simulink library "formationFlyingBlockset"  (R2016b)
settings: Solver=ode45  StartTime=0.0  StopTime=10.0  RelTol=1e-3  EnableMultiTasking=on
undefined symbols (not defined in the file or in its folder): adaptive, aircraftmask_ID, aircraftmask_navigationLaw, aircraftmask_originNED_ECEF_rrm, aircraftmask_p0_NED_m, aircraftmask_phithetapsi_trim, aircraftmask_wakevortexenabled, airkraftmask_displayLeader, DiscIntNeverNeededParam, Earth, fflib_degdegm2rrm, fflib_Hz2radps, fflib_rrm2degdegm, flat2lla, hinf, Klqr, lquadr, mask_ac, mask_ID, mpc, poleplacement, uavsim, washout, WGS84
undefined symbols (not defined in the file): aircraftmask_phithetapsi0, aircraftmask_pqr0, aircraftmask_uvw0, innerloop, outerloop, tatestos
libraries: formationFlyingBlockset x59, aerolibtransform2 x42, simulink_extras x27, dspsrcs4 x11, aerolibutil x5, uavsimBlockset_UAV3DInterface x4, uavsimBlockset_ServoHS55 x4, uavsimBlockset_VectorNorm x3, uavsimBlockset_UAV3DVisualization x3, uavsimBlockset_AugmentWind x3, stringquartett x2, Parrot_DCAS_lib x2
(part 1 of 5)
settings Model: Creator=j.bolting  LastModifiedBy=j.bolting
settings DataIOCC: LimitDataPoints=on  SaveFormat=Array
settings OptimizationCC: ExpressionDepthLimit=2147483647  LifeSpan=inf
settings DebuggingCC: UnderspecifiedInitializationDetection=Classic  MergeDetectMultiDrivingBlocksExec=none  SolverPrmCheckMsg=warning  AllowSymbolicDim=off  StateNameClashWarn=warning  SFUnexpectedBacktrackingDiag=warning  SFNoUnconditionalDefaultTransitionDiag=warning  SFExecutionAtInitializationDiag=none
settings HardwareCC: ProdBitPerPointer=32  ProdBitPerSizeT=32  ProdBitPerPtrDiffT=32  ProdLargestAtomicFloat=None  ProdIntDivRoundTo=Undefined  ProdEndianess=Unspecified  ProdWordSize=32  ProdHWDeviceType=32-bit Generic
settings ModelReferenceCC: PropagateSignalLabelsOutOfModel=off
settings GRTTargetCC: TargetLangStandard=C89/C90 (ANSI)  GeneratePreprocessorConditionals=Disable all
settings ConfigComp: CovMetricSettings=dw  CovHtmlReporting=on  CovSaveCumulativeToWorkspaceVar=on  CovSaveSingleToWorkspaceVar=on  CovExternalEMLEnable=off  CovSFcnEnable=off

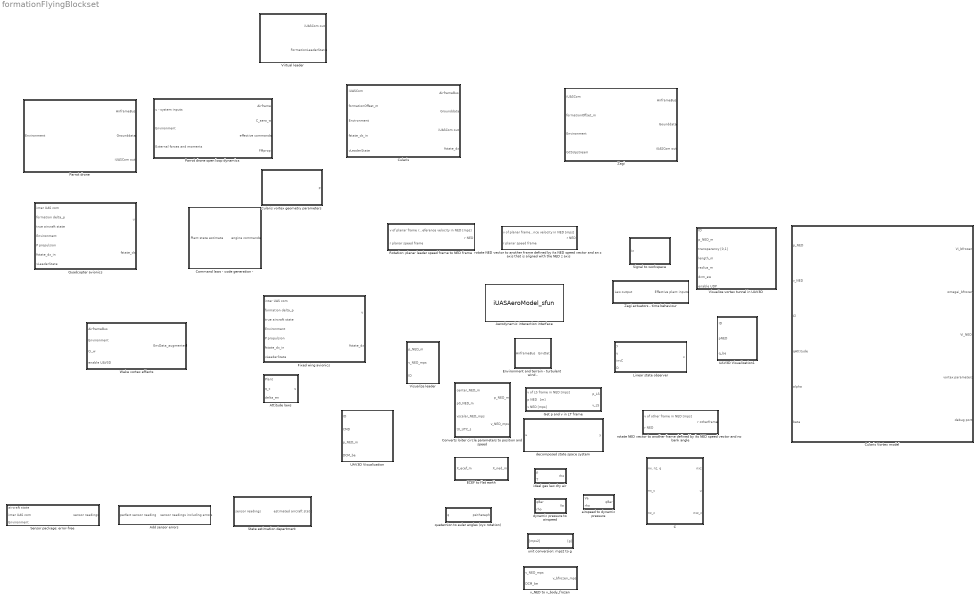
== system formationFlyingBlockset ==
  Add sensor errors : Subsystem
  Aerodynamic interaction interface : M-S-Function  FunctionName=iUASAeroModel_sfun  Parameters=mask_ID, mask_c_m, mask_wingspan_m, mask_sweepangle_rad, mask_dihedral_rad, mask_l_longi_m, mask_nosecoo_m, mask_l_vertical_m, mask_fincoo_m  mask{mask_c_m=0, mask_ID=0, mask_wingspan_m=0, mask_sweepangle_rad=0, mask_dihedral_rad=0, mask_l_longi_m=0, mask_nosecoo_m=0, mask_l_vertical_m=0, mask_fincoo_m=0}
      mask prompts: mask_c_m "Mean aerodynamic chord [m]"; mask_ID "Aircraft ID"; mask_wingspan_m "Wingspan"; mask_sweepangle_rad "Wing sweep angle [rad]"; mask_dihedral_rad "Wing dihedral angle [rad]"; mask_l_longi_m "Longitudinal reference length [m], typically the length of the fuselage"; mask_nosecoo_m "Nose coordinates in the body frame [m m m]"; mask_l_vertical_m "Vertical reference length [m], typically the distance between the lowest point of the fuselage and the tip of the vertical stabilizer"; mask_fincoo_m "Fin tip coordinates in the body frame [m m m]"
      mask help:
      | Interface to the aerodynamic interaction model.
      | This block computes the induced velocities and
      | rotation rates caused by other close UAS and,
      | at the same time, communicates the state of the
      | UAS connected to this block to the aerodynamic
      | interaction model to build a list of all UASs
      | in the airspace.
      mask Display:
      | % Input port names:
      | port_label('input',1,'p{NED}','texmode','on');
      | port_label('input',2,'v{NED}','texmode','on');
      | port_label('input',3,'C_L','texmode','on');
      | port_label('input',4,'q_{Attitude}','texmode','on');
      | port_label('input',5,'[\alpha, \beta]','texmode','on');
      | 
      | % output port names
      | port_label('output',1,'V_{i}^{bfrozen}','texmode','on');
      | port_label('output',2,'\omega_{i}^{bfrozen}','texmode','on');
      | port_label('output',3,'V_i^{NED}','texmode','on');
  Attitude laws : Subsystem  SystemSampleTime=uavsim.ap.hardware.dt_attitudeloops_s
  C : Subsystem
  Command laws - code generation - : Subsystem  TreatAsAtomicUnit=on  SystemSampleTime=0.01
  Converts loiter circle parameters to position and speed : Subsystem
  Cularis : Subsystem  mask{aircraftmask_phithetapsi0=[uavsim.cularis.phithetapsi0(1:2); deg2rad(-30)]', aircraftmask_p0_NED_m=[0 0 -50], aircraftmask_originNED_ECEF_rrm=uavsim.originNED_ECEF_radradm, aircraftmask_pqr0=uavsim.cularis.omega0, aircraftmask_uvw0=uavsim.cularis.uvw0, aircraftmask_phithetapsi_trim=uavsim.cularis.phithetapsi0, aircraftmask_ID=1, aircraftmask_wakevortexenabled=off, aircraftmask_navigationLaw=2, uavsim=uavsim, leaderID=0, airkraftmask_displayLeader=on}
      mask prompts: aircraftmask_phithetapsi0 "Initial Euler angles [rad]"; aircraftmask_p0_NED_m "Initial position, NED frame [m]"; aircraftmask_originNED_ECEF_rrm "Origin NED frame. ECEF, [rad rad m]"; aircraftmask_pqr0 "Initial rotation rates, body frame [rad/s]"; aircraftmask_uvw0 "Initial velocity, body frame [m/s]"; aircraftmask_phithetapsi_trim "Trim Euler angles [rad]"; aircraftmask_ID "Aircraft ID"; aircraftmask_wakevortexenabled "Wake vortex interaction enabled"; aircraftmask_navigationLaw "Active navigation law (-1: automatic selection)"; uavsim "Parameter set"; leaderID "Follows which ID?"; airkraftmask_displayLeader "Display virtual leader"
      mask Display:
      | % Set Icon:
      | image(imread('images/cularis.png'), [.2, .2, .6, .6])
  Cularis Vortex model : Subsystem  mask{mask_ID=aircraftmask_ID}
      mask prompts: mask_ID "ID"
  Cularis vortex geometry parameters : Subsystem  mask{mask_ID=mask_ID}
      mask prompts: mask_ID "ID"
  ECEF to flat earth : Subsystem  mask{mask_originNED_ECEF_rrm=aircraftmask_originNED_ECEF_rrm}
      mask prompts: mask_originNED_ECEF_rrm "Origin NED (lat lon alt [rad, rad, m])"
  Environment and terrain - turbulent wind - : Subsystem  mask{mask_ambientWind=uavsim.environment.ambientWind_NED_mps, mask_wingspan=uavsim.cularis.b, mask_turbulenceON=off, mask_windON=off}
      mask prompts: mask_ambientWind "Ambient wind vector, NED [m/s]"; mask_wingspan "Aircraft wing span [m]"; mask_turbulenceON "Turbulence ON?"; mask_windON "Ambient wind ON?"
  Fixed wing avionics : Subsystem  mask{mask_ac=uavsim.cularis}
      mask prompts: mask_ac "Aircraft specific structure"
      mask Display: image(imread('images/avionics.png'),[.3, .3, .4, .4])
  Get p and v in LT frame : Subsystem
  Linear state observer : Subsystem
  Parrot drone : Subsystem  mask{aircraftmask_phithetapsi0=[uavsim.cularis.phithetapsi0(1:2); deg2rad(-30)]', aircraftmask_p0_NED_m=[0 0 -50], aircraftmask_originNED_ECEF_rrm=uavsim.originNED_ECEF_radradm, aircraftmask_pqr0=uavsim.cularis.omega0, aircraftmask_uvw0=uavsim.cularis.uvw0, aircraftmask_phithetapsi_trim=uavsim.cularis.phithetapsi0, aircraftmask_ID=1, aircraftmask_wakevortexenabled=off, aircraftmask_navigationLaw=2, uavsim=uavsim, leaderID=0, airkraftmask_displayLeader=on}
      mask prompts: aircraftmask_phithetapsi0 "Initial Euler angles [rad]"; aircraftmask_p0_NED_m "Initial position, NED frame [m]"; aircraftmask_originNED_ECEF_rrm "Origin NED frame. ECEF, [rad rad m]"; aircraftmask_pqr0 "Initial rotation rates, body frame [rad/s]"; aircraftmask_uvw0 "Initial velocity, body frame [m/s]"; aircraftmask_phithetapsi_trim "Trim Euler angles [rad]"; aircraftmask_ID "Aircraft ID"; aircraftmask_wakevortexenabled "Wake vortex interaction enabled"; aircraftmask_navigationLaw "Active navigation law (-1: automatic selection)"; uavsim "Parameter set"; leaderID "Follows which ID?"; airkraftmask_displayLeader "Display virtual leader"
      mask Display:
      | % Set Icon:
      | image(imread('images/parrot.png'), [.2, .2, .6, .6])
  Parrot drone open loop dynamics : Subsystem  mask{mask_phithetapsi0=aircraftmask_phithetapsi0, mask_p0_ECEF_lla=fflib_degdegm2rrm(flat2lla(aircraftmask_p0_NED_m, rad2deg(aircraftmask_originNED_ECEF_rrm(1:2)), 0, aircraftmask_originNED_ECEF_rrm(3))), mask_originNED_ECEF_rrm=aircraftmask_originNED_ECEF_rrm, mask_pqr0=aircraftmask_pqr0, mask_uvw0=aircraftmask_uvw0, uavsim=uavsim}
      mask prompts: mask_phithetapsi0 "Initial euler angles [rad]"; mask_p0_ECEF_lla "Initial position ECEF [rad rad m]"; mask_originNED_ECEF_rrm "Origin NED frame, ECEF-WGS84, [rad rad m]"; mask_pqr0 "Initial body rotation rates [rad/s]"; mask_uvw0 "Initial velocity body frame [m/s]"; uavsim "Parameter set"
      mask Display: image(imread('images/parrot.png'),[.3, .3, .4, .4])
  Quadcopter avionics : Subsystem  mask{mask_ac=uavsim.parrot}
      mask prompts: mask_ac "Aircraft specific structure"
      mask Display: image(imread('images/avionics.png'),[.3, .3, .4, .4])
  Rotation: planar leader speed frame to NED frame : Subsystem
  Sensor package: error-free : Subsystem
  Signal to workspace : Subsystem  InitFcn=|  mask{mask_id=['log_ucontroller_UAS' num2str(aircraftmask_ID) '_Signalname'], mask_dt=-1, mask_debug=tatestos}
      | twblock = find_system(gcb, 'LookUnderMasks', 'all' ,'FollowLinks','on', 'BlockType', 'ToWorkspace' );
      | maskblock = find_system(gcb);
      | % Disable library link to be able to modify the block
      | set_param(maskblock{1}, 'LinkStatus', 'inactive');
      | maskparams = get_param(maskblock, 'MaskValues');
      | id = maskparams{1}{3};
      | set_param(twblock{1}, 'VariableName', id);
      | set_param(twblock{1}, 'Name', id);
      mask prompts: mask_id "Variable ID [string, char array], e.g. 'log_voltage'"; mask_dt "Sample time [s]"; mask_debug "debug value"
      mask init:
      | mask_ida = mask_id;
      | mv = get_param(gcb, 'MaskValues');
      | mv{3} = mask_ida;
      | set_param(gcb, 'MaskValues', mv);
      settings: PostSaveFcn=|
      | maskblock = find_system(gcb);
      | set_param(maskblock{1}, 'LinkStatus', 'restore')
      mask Display:
      | % Set Icon:
      | image(imread('images/blocklogo_datalogger.png'))
  State estimation department : Subsystem
  UAV3D Visualization : Subsystem  TreatAsAtomicUnit=on  SystemSampleTime=uavsim.ap.hardware.dt_navigationloops_s  mask{mask_visual=0}
      mask prompts: mask_visual "3D model"
      mask TypeOptions mask_visual: 0 | 1 | 2 | 3
  UAV3D Visualization1 : Subsystem  TreatAsAtomicUnit=on  SystemSampleTime=uavsim.simConfig.tsample_UAV3D  mask{mask_visual=2}
      mask prompts: mask_visual "3D model"
      mask TypeOptions mask_visual: 0 | 1 | 2 | 3
  Virtual leader : Subsystem  mask{aircraftmask_originNED_ECEF_rrm=uavsim.originNED_ECEF_radradm, aircraftmask_ID=0, uavsim=uavsim}
      mask prompts: aircraftmask_originNED_ECEF_rrm "Origin NED frame. ECEF, [rad rad m]"; aircraftmask_ID "Aircraft ID"; uavsim "Parameter set"
      mask Display:
      | % Set Icon:
      | image(imread('images/cularis.png'), [.2, .2, .6, .6])
  Visualize leader : Subsystem  TreatAsAtomicUnit=on  SystemSampleTime=uavsim.simConfig.tsample_UAV3D  mask{mask_3dmodel=1}
      mask prompts: mask_3dmodel "3D model"
      mask TypeOptions mask_3dmodel: 0 | 1 | 2 | 3
  Visualize vortex tunnel in UAV3D : Subsystem  TreatAsAtomicUnit=on  SystemSampleTime=uavsim.simConfig.tsample_UAV3D
  Wake vortex effects : Subsystem  TreatAsAtomicUnit=on
  Zagi : Subsystem  mask{aircraftmask_phithetapsi0=[uavsim.zagi.phithetapsi0(1:2); deg2rad(30)]', aircraftmask_p0_NED_m=[0 0 -50], aircraftmask_originNED_ECEF_rrm=uavsim.originNED_ECEF_radradm, aircraftmask_pqr0=uavsim.zagi.omega0, aircraftmask_uvw0=uavsim.zagi.uvw0, aircraftmask_phithetapsi_trim=uavsim.zagi.phithetapsi0, aircraftmask_ID=1, aircraftmask_wakevortexenabled=off, aircraftmask_navigationLaw=3, uavsim=uavsim, leaderID=0}
      mask prompts: aircraftmask_phithetapsi0 "Initial Euler angles [rad]"; aircraftmask_p0_NED_m "Initial position, NED frame [m]"; aircraftmask_originNED_ECEF_rrm "Origin NED frame. ECEF, [rad rad m]"; aircraftmask_pqr0 "Initial rotation rates, body frame [rad/s]"; aircraftmask_uvw0 "Initial velocity, body frame [m/s]"; aircraftmask_phithetapsi_trim "Trim Euler angles [rad]"; aircraftmask_ID "Aircraft ID"; aircraftmask_wakevortexenabled "Wake vortex interaction enabled"; aircraftmask_navigationLaw "Active navigation law (-1: automatic selection)"; uavsim "Parameter set"; leaderID "Follows which ID?"
      mask Display:
      | % Set Icon:
      | image(imread('images/zagi_slope.png'))
      | %image(imread('images/aerosonde_MKII.png'),[.2, .2, .6, .6])
      | % Port labels:
      | port_label('input',1,'Com_{interUAS}','texmode','on');
      | port_label('input',2,'offset_{formation}','texmode','on');
      | port_label('input',3,'Environment','texmode','on');
      | port_label('input',4,'GCS_{Upstream}','texmode','on');
      | 
      | port_label('output',1,'Airframe_{Bus}','texmode','on');
      | port_label('output',2,'GroundData','texmode','on');
      | port_label('output',3,'iUAS_{Com}','texmode','on');
  Zagi actuators - time behaviour : Subsystem  TreatAsAtomicUnit=on
  airspeed to dynamic pressure : Subsystem
  decomposed state space system : Subsystem  mask{ss_innerloop=innerloop, ss_outerloop=outerloop}
      mask prompts: ss_innerloop "State space model inner loop"; ss_outerloop "State space model outer loop"
  dynamic pressure to airspeed : Subsystem
  ideal gas law dry air : Subsystem
  quaternion to euler angles (zyx rotation) : Subsystem
  rotate NED vector to another frame defined by its NED speed vector and an z axis that is aligned with the NED z axis : Subsystem
  rotate NED vector to another frame defined by its NED speed vector and no bank angle : Subsystem
  unit conversion: mps2 to g : Subsystem
  v_NED to v_body_frozen : Subsystem

== system formationFlyingBlockset/Add sensor errors ==
  perfect sensor reading : Inport  OutDataTypeStr=Bus: SensorBus
  AHRS : Subsystem
  Air Data : Subsystem
  Bus Object Bus Creator : BusCreator  Inputs=8  OutDataTypeStr=Bus: SensorBus  mask(BUS OBJECT Bus Creator){busType=Bus: SensorBus}
      mask prompts: busType "Bus Type"
      mask help:
      | Provides users the cabability to painlessly, instantly customize bus creators of output data type 'Bus:' by selecting the bus object type from a drop down menu dynamically populated by bus objects in the workspace.
      |
      | After pressing the "Apply Selection" button signal lines into the creator are populated and named with the elements in the chosen bus saving the user from having to recall and fill out signal line names.
      |
      | NOTE that when copying a Bus Object Bus Creator from your locked Library the link to the Library is automatically broken. This saves the user from having to Unlock Links To Library (From the Library menu.), Disable Link and finally Break Link (Both from the Model menu.) for every placed instance of the block.
      settings: AttributesFormatString=%<OutDataTypeStr>  CopyFcn=set_param(gcb, 'LinkStatus', 'none')
      mask TypeOptions busType: Bus: AHRS | Bus: Acceleration | Bus: Aero | Bus: Airdata | Bus: Airframe | Bus: Attitude | Bus: CMD | Bus: CMD_quadrotor | Bus: ControlInfoBus | Bus: Enginedata | Bus: Environment | Bus: FlightGearData | Bus: GCSUpstream | Bus: GNSSL1 | Bus: GNSSRTK | Bus: GPS | Bus: IMU | Bus: Kinematics | Bus: LandinggearInput | Bus: MotionTracker | Bus: Position | Bus: Radiodistance | Bus: RotationalAcceleration | Bus: RotationalVelocity | Bus: SensorBus | Bus: StateBus | Bus: Velocity | Bus: WindAngles | Bus: iUAScom
      mask Callback busType:
      | % Using variable names terminated with "_BOBC" to lessen the chances of
      | % collisions with existing workspace variables.
      | 
      | % Get the current block handle and mask handle.
      | handleCreator_BOBC = gcbh;
      | maskObj_BOBC       = Simulink.Mask.get(gcb);
      | 
      | % Get a list of variables in the workspace in order to search for the '1x1
      | % Bus' types.
      | wsVars_BOBC = whos;
      | 
      | % Reset the 'TypeOptions' bus list in case some '1x1 Bus' types have been
      | % deleted from or added to the workspace.
      | maskObj_BOBC.Parameters.TypeOptions = {'<empty>'};
      | 
      | % Reset the bus count.
      | busCount_BOBC = 0;
      | 
      | for index_BOBC = 1:length(wsVars_BOBC)
      | 
      |    % If the variable is a bus object...
      |    if strcmp(wsVars_BOBC(index_BOBC).class, 'Simulink.Bus')
      | 
      |       busCount_BOBC = busCount_BOBC + 1;
      | 
      |       % ... add it to the TypeOptions of the mask.
      |       maskObj_BOBC.Parameters.TypeOptions(busCount_BOBC) = ...
      |                                                            ...
      |                                  {['Bus: ', wsVars_BOBC(index_BOBC).name]};
      |    end
      | end
      | 
      | if busCount_BOBC == 0
      | 
      |    % If there are NO bus objects in the workspace then provide a warning
      |    % popup...
      |    warndlg('There are currently no bus objects in the workspace - you have no use for this block. Use a normal Bus Creator instead.')
      | 
      |    % ... and do nothing.
      | elseif ~strcmp(get_param(handleCreator_BOBC, 'OutDataTypeStr'), 'Inherit: auto')
      | 
      |    % If the currently selected bus data type ('OutDataTypeStr') is not
      |    % 'Inherit: auto' (i.e., if we are reopening the mask.) then get the
      |    % current 'OutDataTypeStr' and 'maskVal.' ('maskVal' is the selected
      |    % 'TypeOptions' list member.)
      |    outDatStr_BOBC = get_param(handleCreator_BOBC, 'OutDataTypeStr');
      |    maskVal_BOBC   = get_param(handleCreator_BOBC, 'MaskValues');
      | 
      |    if ~strcmp(outDatStr_BOBC, maskVal_BOBC{1})
      | 
      |       % Upon re-opening the mask if the default 'TypeOptions' list member
      |       % (The first one.) contained in 'maskVal' does not match the
      |       % currently selected bus data type ('OutDataTypeStr') then set the
      |       % 'TypeOptions' list member to the selected bus data type. (Cuts down
      |       % on confusion to have the displayed list member match the selected
      |       % bus data type rather than the first entry.)
      |       set_param(handleCreator_BOBC, 'MaskValues', {outDatStr_BOBC});
      |    end
      | end
      | 
      | % Clean up the workspace.
      | clear  handleCreator_BOBC  maskObj_BOBC     wsVars_BOBC ...
      |             busCount_BOBC    index_BOBC  outDatStr_BOBC ...
      |              maskVal_BOBC
      mask DialogControl applyMOCBSelection Prompt: Apply Selection
      mask DialogControl applyMOCBSelection Callback:
      | % Using variable names terminated with "_BOBC" to lessen the chances of
      | % collisions with existing workspace variables.
      | 
      | % Get the current block, current block handle and mask handle.
      | currentBlock_BOBC  = gcb;
      | handleCreator_BOBC = gcbh;
      | 
      | % Get the desired bus type...
      | desiredBusType_BOBC = get_param(handleCreator_BOBC, 'busType');
      | 
      | % ... and set the 'OutDataTypeStr' to it.
      | set_param(handleCreator_BOBC, 'OutDataTypeStr', desiredBusType_BOBC);
      | 
      | %% First delete any existing lines on the port.
      | % Get the line handles.
      | lh_BOBC = get_param(handleCreator_BOBC, 'LineHandles');
      | 
      | % If any lines exist (Non- -1 line handles.), delete them and start over.
      | if max(lh_BOBC.Inport > 0)
      | 
      |    for index_BOBC = 1:length(lh_BOBC.Inport)
      | 
      |       if lh_BOBC.Inport(index_BOBC) > 0
      | 
      |          delete_line(lh_BOBC.Inport(index_BOBC))
      |       end
      |    end
      | end
      | 
      | %% Then work on adding new lines.
      | 
      | % Get the block path for 'add_line' function.
      | blockPath_BOBC = get_param(handleCreator_BOBC, 'Parent');
      | 
      | % Get the newly selected bus type ('OutDataTypeStr')...
      | mocbBusType_BOBC = get_param(currentBlock_BOBC, 'OutDataTypeStr');
      | 
      | % ... and parse off "Bus: " so the string of the desired bus contained in
      | % 'OutDataTypeStr' matches the raw workspace bus names.
      | mocbBusType_BOBC = mocbBusType_BOBC(6:end);
      | 
      | % Then evaluate the string containing the workspace bus name which will
      | % load the desired bus parameters.
      | busParams_BOBC = eval(mocbBusType_BOBC);
      | 
      | % From the parameters grab the number of lines to add.
      | numLines_BOBC = length(busParams_BOBC.Elements);
      | 
      | % Set the number of inputs of the masked bus creator to the number of lines
      | % to add.
      | set_param(handleCreator_BOBC, 'Inputs', num2str(numLines_BOBC));
      | 
      | % Get (Inputs.) port handles so we can grab the positions of them.
      | ph_BOBC = get_param(handleCreator_BOBC, 'PortHandles');
      | 
      | for index_BOBC = 1:numLines_BOBC
      | 
      |    % Get the position of input port number 'index_BOBC'.
      |    portPos_BOBC = get_param(ph_BOBC.Inport(index_BOBC), 'Position');
      | 
      |    % Add a line from 50 pixels left of the port position to the port
      |    % position. (This must be done because it's the lines that get named,
      |    % not the port positions.)
      |    portLine_BOBC = add_line(blockPath_BOBC, [portPos_BOBC - [50 0]; portPos_BOBC]);
      | 
      |    % Rename the new line to the bus 'index_BOBC-st/nd/rd/th' element name.
      |    set_param(portLine_BOBC, 'Name', busParams_BOBC.Elements(index_BOBC).Name)
      | end
      | 
      | %% Cleanup the workspace.
      | clear    currentBlock_BOBC  handleCreator_BOBC      index_BOBC ...
      |        desiredBusType_BOBC             lh_BOBC  blockPath_BOBC ...
      |           mocbBusType_BOBC      busParams_BOBC   numLines_BOBC ...
      |                    ph_BOBC        portPos_BOBC   portLine_BOBC
  L1 GPS : Subsystem
  Optitrack : Subsystem
  Propulsion sensors : Subsystem
  RTK DGPS : Subsystem
  Radio distance sensor : Subsystem
  Wind angle sensors : Subsystem
  sensor readings including errors : Outport  OutDataTypeStr=Bus: SensorBus
  wires:
  Bus Object Bus Creator/1 -> sensor readings including errors/1
  perfect sensor reading/1 -> AHRS/1(perfect sensor reading), RTK DGPS/1(perfect sensor reading), L1 GPS/1(perfect sensor reading), Optitrack/1(perfect sensor reading), Propulsion sensors/1(perfect sensor reading), Radio distance sensor/1(perfect sensor reading), Wind angle sensors/1(perfect sensor reading), Air Data/1(perfect sensor reading)
  AHRS/1(output) -> Bus Object Bus Creator/1  "ahrs"
  Air Data/1(output) -> Bus Object Bus Creator/2  "airdata"
  L1 GPS/1(output) -> Bus Object Bus Creator/3  "gnss_l1"
  RTK DGPS/1(output) -> Bus Object Bus Creator/4  "gnss_rtk"
  Propulsion sensors/1(output) -> Bus Object Bus Creator/5  "propulsion"
  Radio distance sensor/1(output) -> Bus Object Bus Creator/6  "radiodistance"
  Wind angle sensors/1(output) -> Bus Object Bus Creator/7  "windangles"
  Optitrack/1(output) -> Bus Object Bus Creator/8  "motiontracker"

== system formationFlyingBlockset/Attitude laws ==
  Plant : Inport  OutDataTypeStr=Bus: StateBus
  q_c : Inport  Port=2
  delta_en : Inport  Port=3
  Add : Sum
  Add1 : Sum
  Bus Creator2 : BusCreator  Inputs=5  OutDataTypeStr=Bus: CMD  NonVirtualBus=on
  Constant : Constant  Value=zeros(3,1)
  Demux : Demux
  Local rotation angle attitude control : Subsystem
  Mux : Mux  Inputs=2
  Saturation : Saturate  UpperLimit=1  LowerLimit=0
  Trim Inputs : Constant  Value=[mask_ac.u_trim(1:4)]
  no flaps : Constant  Value=0
  u : Outport  OutDataTypeStr=Bus: CMD
  wires:
  Demux/4 -> Saturation/1  "den_0to1"
  Local rotation angle attitude control/1(u) -> Add1/1
  Bus Creator2/1 -> u/1  "CMD"
  Demux/3 -> Bus Creator2/3  "dr_rad"
  Saturation/1 -> Bus Creator2/4  "den_0to1"
  Demux/1 -> Bus Creator2/1  "da_rad"
  Demux/2 -> Bus Creator2/2  "de_rad"
  Trim Inputs/1 -> Add/1
  Add/1 -> Demux/1
  Plant/1 -> Local rotation angle attitude control/1(Plant)
  q_c/1 -> Local rotation angle attitude control/2(q_c)
  Constant/1 -> Mux/1
  Mux/1 -> Add1/2
  Add1/1 -> Add/2
  delta_en/1 -> Mux/2
  no flaps/1 -> Bus Creator2/5  "df_rad"

== system formationFlyingBlockset/C ==
  "nx, nz, q" : Inport
  nx_c : Inport  Port=2
  nz_c : Inport  Port=3
  Gain1 : Gain  Gain=Klqr  Multiplication=Matrix(K*u)
  Integrator : Integrator
  Integrator1 : Integrator
  Mux1 : Mux  Inputs=3
  Mux2 : Mux  Inputs=2
  Mux5 : Mux  Inputs=2
  Sum : Sum  Inputs=|+-
  get n_xz : Selector  InputPortWidth=3  IndexOptions=Index vector (dialog)  Indices=1:2  OutputSizes=1
  get q : Selector  InputPortWidth=3  IndexOptions=Index vector (dialog)  Indices=3  OutputSizes=1
  nxz : Outport
  u : Outport  Port=2
  nxz_c : Outport  Port=3
  wires:
  Integrator1/1 -> Mux1/3  "integrated load factor errors"
  nz_c/1 -> Mux2/2
  get q/1 -> Mux5/2
  nx_c/1 -> Mux2/1
  get n_xz/1 -> Sum/1, nxz/1
  Mux2/1 -> Sum/2, nxz_c/1
  Mux5/1 -> Mux1/1
  Sum/1 -> Mux5/1, Integrator1/1  "load factor errors"
  "nx, nz, q"/1 -> get q/1, get n_xz/1
  Gain1/1 -> Integrator/1
  Integrator/1 -> Mux1/2, u/1
  Mux1/1 -> Gain1/1

== system formationFlyingBlockset/Command laws - code generation - ==
  Plant state estimate : Inport  OutDataTypeStr=Bus: StateBus
  Add : Sum  Inputs=+++
  Bus Object Bus Creator : BusCreator  Inputs=1  OutDataTypeStr=Bus: CMD_quadrotor  mask(BUS OBJECT Bus Creator){busType=Bus: CMD_quadrotor}
      mask prompts: busType "Bus Type"
      mask help:
      | Provides users the cabability to painlessly, instantly customize bus creators of output data type 'Bus:' by selecting the bus object type from a drop down menu dynamically populated by bus objects in the workspace.
      |
      | After pressing the "Apply Selection" button signal lines into the creator are populated and named with the elements in the chosen bus saving the user from having to recall and fill out signal line names.
      |
      | NOTE that when copying a Bus Object Bus Creator from your locked Library the link to the Library is automatically broken. This saves the user from having to Unlock Links To Library (From the Library menu.), Disable Link and finally Break Link (Both from the Model menu.) for every placed instance of the block.
      settings: AttributesFormatString=%<OutDataTypeStr>  CopyFcn=set_param(gcb, 'LinkStatus', 'none')
      mask TypeOptions busType: Bus: AHRS | Bus: Acceleration | Bus: Aero | Bus: Airdata | Bus: Airframe | Bus: Attitude | Bus: CMD | Bus: CMD_quadrotor | Bus: ControlInfoBus | Bus: Enginedata | Bus: Environment | Bus: FlightGearData | Bus: GCSUpstream | Bus: GNSSL1 | Bus: GNSSRTK | Bus: GPS | Bus: IMU | Bus: Kinematics | Bus: LandinggearInput | Bus: MotionTracker | Bus: Position | Bus: Radiodistance | Bus: RotationalAcceleration | Bus: RotationalVelocity | Bus: SensorBus | Bus: StateBus | Bus: Velocity | Bus: WindAngles | Bus: iUAScom
      mask Callback busType:
      | % Using variable names terminated with "_BOBC" to lessen the chances of
      | % collisions with existing workspace variables.
      | 
      | % Get the current block handle and mask handle.
      | handleCreator_BOBC = gcbh;
      | maskObj_BOBC       = Simulink.Mask.get(gcb);
      | 
      | % Get a list of variables in the workspace in order to search for the '1x1
      | % Bus' types.
      | wsVars_BOBC = whos;
      | 
      | % Reset the 'TypeOptions' bus list in case some '1x1 Bus' types have been
      | % deleted from or added to the workspace.
      | maskObj_BOBC.Parameters.TypeOptions = {'<empty>'};
      | 
      | % Reset the bus count.
      | busCount_BOBC = 0;
      | 
      | for index_BOBC = 1:length(wsVars_BOBC)
      | 
      |    % If the variable is a bus object...
      |    if strcmp(wsVars_BOBC(index_BOBC).class, 'Simulink.Bus')
      | 
      |       busCount_BOBC = busCount_BOBC + 1;
      | 
      |       % ... add it to the TypeOptions of the mask.
      |       maskObj_BOBC.Parameters.TypeOptions(busCount_BOBC) = ...
      |                                                            ...
      |                                  {['Bus: ', wsVars_BOBC(index_BOBC).name]};
      |    end
      | end
      | 
      | if busCount_BOBC == 0
      | 
      |    % If there are NO bus objects in the workspace then provide a warning
      |    % popup...
      |    warndlg('There are currently no bus objects in the workspace - you have no use for this block. Use a normal Bus Creator instead.')
      | 
      |    % ... and do nothing.
      | elseif ~strcmp(get_param(handleCreator_BOBC, 'OutDataTypeStr'), 'Inherit: auto')
      | 
      |    % If the currently selected bus data type ('OutDataTypeStr') is not
      |    % 'Inherit: auto' (i.e., if we are reopening the mask.) then get the
      |    % current 'OutDataTypeStr' and 'maskVal.' ('maskVal' is the selected
      |    % 'TypeOptions' list member.)
      |    outDatStr_BOBC = get_param(handleCreator_BOBC, 'OutDataTypeStr');
      |    maskVal_BOBC   = get_param(handleCreator_BOBC, 'MaskValues');
      | 
      |    if ~strcmp(outDatStr_BOBC, maskVal_BOBC{1})
      | 
      |       % Upon re-opening the mask if the default 'TypeOptions' list member
      |       % (The first one.) contained in 'maskVal' does not match the
      |       % currently selected bus data type ('OutDataTypeStr') then set the
      |       % 'TypeOptions' list member to the selected bus data type. (Cuts down
      |       % on confusion to have the displayed list member match the selected
      |       % bus data type rather than the first entry.)
      |       set_param(handleCreator_BOBC, 'MaskValues', {outDatStr_BOBC});
      |    end
      | end
      | 
      | % Clean up the workspace.
      | clear  handleCreator_BOBC  maskObj_BOBC     wsVars_BOBC ...
      |             busCount_BOBC    index_BOBC  outDatStr_BOBC ...
      |              maskVal_BOBC
      mask DialogControl applyMOCBSelection Prompt: Apply Selection
      mask DialogControl applyMOCBSelection Callback:
      | % Using variable names terminated with "_BOBC" to lessen the chances of
      | % collisions with existing workspace variables.
      | 
      | % Get the current block, current block handle and mask handle.
      | currentBlock_BOBC  = gcb;
      | handleCreator_BOBC = gcbh;
      | 
      | % Get the desired bus type...
      | desiredBusType_BOBC = get_param(handleCreator_BOBC, 'busType');
      | 
      | % ... and set the 'OutDataTypeStr' to it.
      | set_param(handleCreator_BOBC, 'OutDataTypeStr', desiredBusType_BOBC);
      | 
      | %% First delete any existing lines on the port.
      | % Get the line handles.
      | lh_BOBC = get_param(handleCreator_BOBC, 'LineHandles');
      | 
      | % If any lines exist (Non- -1 line handles.), delete them and start over.
      | if max(lh_BOBC.Inport > 0)
      | 
      |    for index_BOBC = 1:length(lh_BOBC.Inport)
      | 
      |       if lh_BOBC.Inport(index_BOBC) > 0
      | 
      |          delete_line(lh_BOBC.Inport(index_BOBC))
      |       end
      |    end
      | end
      | 
      | %% Then work on adding new lines.
      | 
      | % Get the block path for 'add_line' function.
      | blockPath_BOBC = get_param(handleCreator_BOBC, 'Parent');
      | 
      | % Get the newly selected bus type ('OutDataTypeStr')...
      | mocbBusType_BOBC = get_param(currentBlock_BOBC, 'OutDataTypeStr');
      | 
      | % ... and parse off "Bus: " so the string of the desired bus contained in
      | % 'OutDataTypeStr' matches the raw workspace bus names.
      | mocbBusType_BOBC = mocbBusType_BOBC(6:end);
      | 
      | % Then evaluate the string containing the workspace bus name which will
      | % load the desired bus parameters.
      | busParams_BOBC = eval(mocbBusType_BOBC);
      | 
      | % From the parameters grab the number of lines to add.
      | numLines_BOBC = length(busParams_BOBC.Elements);
      | 
      | % Set the number of inputs of the masked bus creator to the number of lines
      | % to add.
      | set_param(handleCreator_BOBC, 'Inputs', num2str(numLines_BOBC));
      | 
      | % Get (Inputs.) port handles so we can grab the positions of them.
      | ph_BOBC = get_param(handleCreator_BOBC, 'PortHandles');
      | 
      | for index_BOBC = 1:numLines_BOBC
      | 
      |    % Get the position of input port number 'index_BOBC'.
      |    portPos_BOBC = get_param(ph_BOBC.Inport(index_BOBC), 'Position');
      | 
      |    % Add a line from 50 pixels left of the port position to the port
      |    % position. (This must be done because it's the lines that get named,
      |    % not the port positions.)
      |    portLine_BOBC = add_line(blockPath_BOBC, [portPos_BOBC - [50 0]; portPos_BOBC]);
      | 
      |    % Rename the new line to the bus 'index_BOBC-st/nd/rd/th' element name.
      |    set_param(portLine_BOBC, 'Name', busParams_BOBC.Elements(index_BOBC).Name)
      | end
      | 
      | %% Cleanup the workspace.
      | clear    currentBlock_BOBC  handleCreator_BOBC      index_BOBC ...
      |        desiredBusType_BOBC             lh_BOBC  blockPath_BOBC ...
      |           mocbBusType_BOBC      busParams_BOBC   numLines_BOBC ...
      |                    ph_BOBC        portPos_BOBC   portLine_BOBC
  Hover input : Constant  Value=uavsim.parrot.u0
  LQR altitude : Subsystem
  LQR attitude : Subsystem
  LQR roll & pitch : Subsystem
  Saturation : Saturate  UpperLimit=ones(4,1)  LowerLimit=zeros(4,1)
  Scope : Scope
  engine commands : Outport  OutDataTypeStr=Bus: CMD_quadrotor
  wires:
  Add/1 -> Scope/1, Bus Object Bus Creator/1  "cmd_engine_0t01"
  Plant state estimate/1 -> LQR attitude/1(State estimate), LQR altitude/1(State estimate), LQR roll & pitch/1(State estimate)
  Bus Object Bus Creator/1 -> engine commands/1
  Hover input/1 -> Add/1
  LQR roll & pitch/1(u) -> ?
  LQR altitude/1(u) -> Add/2
  LQR attitude/1(u) -> Add/3

== system formationFlyingBlockset/Converts loiter circle parameters to position and speed ==
  center_NED_m : Inport
  p0_NED_m : Inport  Port=2
  vscalar_NED_mps : Inport  Port=3
  t0_UTC_s : Inport  Port=4
  3x3 Cross Product : aerolibutil/3x3 Cross Product
  Add : Sum
  Add1 : Sum  Inputs=-+
  Add2 : Sum  Inputs=-+
  Constant : Constant  Value=[0 0]
  Constant1 : Constant  Value=[0 0 1]'  VectorParams1D=off
  Divide flown distance by circle perimeter1 : Product  Inputs=/*
  Gain : Gain  Gain=-1
  Matrix Multiply : Product  Multiplication=Matrix(*)
  Mux : Mux  Inputs=2
  Product : Product  RndMeth=Zero
  Product1 : Product  RndMeth=Zero
  Rotation Angles to Direction Cosine Matrix : aerolibtransform2/Rotation Angles to Direction Cosine Matrix  rotationOrder=ZYX
  UTC_s : Clock
      settings: Decimation=3
  unit vector : uavsimBlockset_UnitVector/unit vector
  vector norm : uavsimBlockset_VectorNorm/vector norm
  p_NED_m : Outport
  v_NED_mps : Outport  Port=2
  wires:
  center_NED_m/1 -> Add2/1, Add/1
  Add/1 -> p_NED_m/1
  UTC_s/1 -> Add1/2
  t0_UTC_s/1 -> Add1/1
  Add1/1 -> Product/2  "time since t0"
  p0_NED_m/1 -> Add2/2
  Add2/1 -> Matrix Multiply/2, vector norm/1  "initial radius vector"
  vector norm/1 -> Divide flown distance by circle perimeter1/1  "r"
  Divide flown distance by circle perimeter1/1 -> Product/1  "psiDot"
  Product/1 -> Mux/1
  Mux/1 -> Rotation Angles to Direction Cosine Matrix/1
  Constant/1 -> Mux/2
  Rotation Angles to Direction Cosine Matrix/1 -> Matrix Multiply/1
  Matrix Multiply/1 -> Add/2, 3x3 Cross Product/2
  3x3 Cross Product/1 -> unit vector/1
  vscalar_NED_mps/1 -> Product1/1, Divide flown distance by circle perimeter1/2
  Product1/1 -> Gain/1
  unit vector/1 -> Product1/2
  Constant1/1 -> 3x3 Cross Product/1
  Gain/1 -> v_NED_mps/1

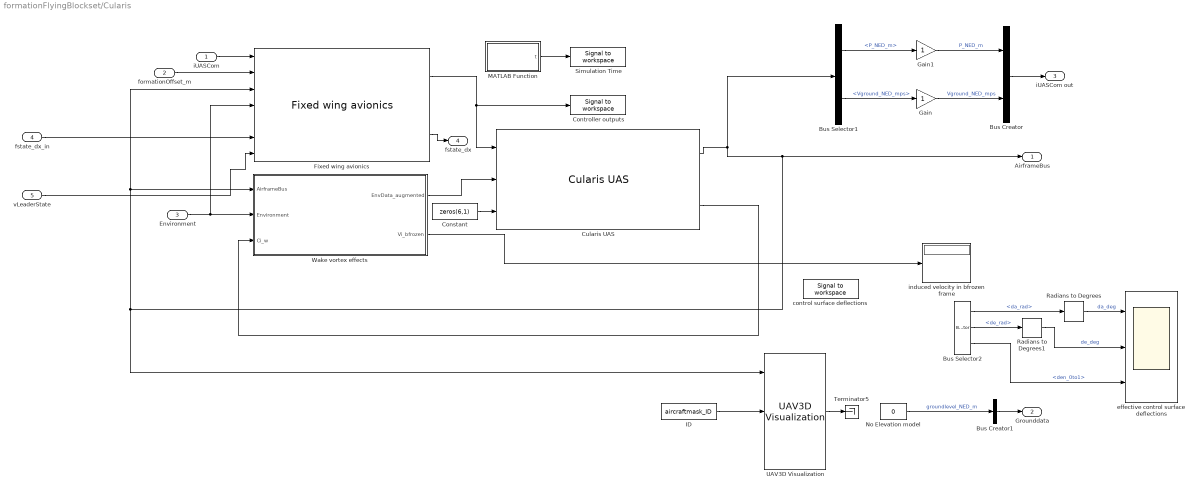
== system formationFlyingBlockset/Cularis ==
  iUASCom : Inport  OutDataTypeStr=Bus: iUAScom
  formationOffset_m : Inport  Port=2
  Environment : Inport  Port=3  OutDataTypeStr=Bus: Environment
  fstate_dx_in : Inport  Port=4
  vLeaderState : Inport  Port=5  OutDataTypeStr=Bus: iUAScom
  Bus Creator : BusCreator  Inputs=2  OutDataTypeStr=Bus: iUAScom
  Bus Creator1 : BusCreator  Inputs=1  OutDataTypeStr=Bus: FlightGearData  NonVirtualBus=on
  Bus Selector1 : BusSelector  OutputSignals=Kinematics.Position.P_NED_m,Kinematics.Velocity.Vground_NED_mps
  Bus Selector2 : BusSelector  OutputSignals=da_rad,de_rad,den_0to1
  Constant : Constant  Value=zeros(6,1)
  Controller outputs : formationFlyingBlockset/Signal to workspace  mask_id=['log_ucontroller_UAS' num2str(aircraftmask_ID) ]  mask_dt=0.01  mask_debug=log_ucontroller_UAS1
  Cularis UAS : uavsimblockset/Cularis UAS  mask_cularis_phithetapsi0=aircraftmask_phithetapsi0  mask_cularis_p0_ECEF_lla=fflib_degdegm2rrm(flat2lla(aircraftmask_p0_NED_m, rad2deg(aircraftmask_originNED_ECEF_rrm(1:2)), 0, aircraftmask_originNED_ECEF_rrm(3)))  mask_cularis_originNED_ECEF_rrm=aircraftmask_originNED_ECEF_rrm  mask_cularis_pqr0=aircraftmask_pqr0  mask_cularis_uvw0=aircraftmask_uvw0  uavsim=uavsim
      link override Cularis actuators - time behaviour/Servo HS1: SourceBlock=uavsimBlockset_ServoHS55/Servo HS55  mask_initialPosition=uavsim.cularis.u0.de
      link override Cularis actuators - time behaviour/Servo HS2: SourceBlock=uavsimBlockset_ServoHS55/Servo HS55  mask_initialPosition=uavsim.cularis.u0.dr
      link override Cularis actuators - time behaviour/Servo HS3: SourceBlock=uavsimBlockset_ServoHS55/Servo HS55  mask_initialPosition=uavsim.cularis.u0.df
      link override Cularis actuators - time behaviour/Servo HS55: SourceBlock=uavsimBlockset_ServoHS55/Servo HS55  mask_initialPosition=uavsim.cularis.u0.da
  Fixed wing avionics : formationFlyingBlockset/Fixed wing avionics  mask_ac=uavsim.cularis
  Gain : Gain
  Gain1 : Gain
  ID : Constant  Value=aircraftmask_ID
  MATLAB Function : MATLAB Function  TreatAsAtomicUnit=on
  No Elevation model : Constant  Value=0
  Radians to Degrees : simulink_extras/Transformations/Radians to Degrees
  Radians to Degrees1 : simulink_extras/Transformations/Radians to Degrees
  Simulation Time : formationFlyingBlockset/Signal to workspace  mask_id=['log_machinetime_UAS' num2str(aircraftmask_ID) ]  mask_dt=1  mask_debug=log_machinetime_UAS1
  Terminator5 : Terminator
  UAV3D Visualization : uavsimBlockset_UAV3DVisualization/UAV3D Visualization  mask_visual=2
  Wake vortex effects : Subsystem  TreatAsAtomicUnit=on
  control surface deflections : formationFlyingBlockset/Signal to workspace  mask_id=['log_csdeflct_UAS' num2str(aircraftmask_ID) ]  mask_dt=-1  mask_debug=log_csdeflct_UAS1
  effective control surface deflections : Scope  NumInputPorts=3
  induced velocity in bfrozen frame : Display
  AirframeBus : Outport
  Grounddata : Outport  Port=2  OutDataTypeStr=Bus: FlightGearData
  iUASCom out : Outport  Port=3
  fstate_dx : Outport  Port=4
  wires:
  vLeaderState/1 -> Fixed wing avionics/7
  Bus Selector2/3 -> effective control surface deflections/3  "<den_0to1>"
  Radians to Degrees1/1 -> effective control surface deflections/2  "de_deg"
  Radians to Degrees/1 -> effective control surface deflections/1  "da_deg"
  Fixed wing avionics/1 -> Controller outputs/1, Cularis UAS/1
  formationOffset_m/1 -> Fixed wing avionics/2
  iUASCom/1 -> Fixed wing avionics/1
  UAV3D Visualization/1 -> Terminator5/1
  No Elevation model/1 -> Bus Creator1/1  "groundlevel_NED_m"
  Bus Creator1/1 -> Grounddata/1
  Bus Selector2/2 -> Radians to Degrees1/1  "<de_rad>"
  Bus Selector2/1 -> Radians to Degrees/1  "<da_rad>"
  ID/1 -> UAV3D Visualization/2
  Wake vortex effects/1(EnvData_augmented) -> Cularis UAS/2
  Wake vortex effects/2(Vi_bfrozen) -> induced velocity in bfrozen frame/1
  Cularis UAS/2 -> Wake vortex effects/3(Ci_w)
  Environment/1 -> Wake vortex effects/2(Environment), Fixed wing avionics/4
  Cularis UAS/1 -> Wake vortex effects/1(AirframeBus), Fixed wing avionics/3, UAV3D Visualization/1, AirframeBus/1, Bus Selector1/1
  ? -> Bus Selector2/1, UAV3D Visualization/3, control surface deflections/1
  Constant/1 -> Cularis UAS/3
  Gain/1 -> Bus Creator/2  "Vground_NED_mps"
  Gain1/1 -> Bus Creator/1  "P_NED_m"
  Bus Selector1/1 -> Gain1/1  "<P_NED_m>"
  Bus Selector1/2 -> Gain/1  "<Vground_NED_mps>"
  Bus Creator/1 -> iUASCom out/1
  Fixed wing avionics/2 -> fstate_dx/1
  fstate_dx_in/1 -> Fixed wing avionics/6
  MATLAB Function/1(t) -> Simulation Time/1

== system formationFlyingBlockset/Cularis Vortex model ==
  p_NED : Inport
  v_NED : Inport  Port=2
  Cl : Inport  Port=3
  qAttitude : Inport  Port=4
  alpha : Inport  Port=5
  beta : Inport  Port=6
  Bus Creator : BusCreator  Inputs=3
  Clock : Clock
  Cularis vortex geometry parameters : formationFlyingBlockset/Cularis vortex geometry parameters  mask_ID=mask_ID
  Display : Display
  MATLAB Function1 : MATLAB Function  TreatAsAtomicUnit=on
  Signal Conversion : SignalConversion  OverrideOpt=off
  Vi_bfrozen : Outport
  omegai_bfrozen : Outport  Port=2
  Vi_NED : Outport  Port=3
  vortex parameters : Outport  Port=4
  debug port : Outport  Port=5
  wires:
  MATLAB Function1/7(debugport) -> debug port/1
  MATLAB Function1/3(Vi_NED) -> Vi_NED/1
  beta/1 -> MATLAB Function1/6(beta)
  alpha/1 -> MATLAB Function1/5(alpha)
  qAttitude/1 -> MATLAB Function1/4(qAttitude)
  Cl/1 -> MATLAB Function1/3(CL)
  v_NED/1 -> MATLAB Function1/2(vNED)
  p_NED/1 -> MATLAB Function1/1(pNED)
  Cularis vortex geometry parameters/1 -> MATLAB Function1/7(p)
  Clock/1 -> MATLAB Function1/8(tsim)
  MATLAB Function1/1(Vi_bfrozen) -> Vi_bfrozen/1
  MATLAB Function1/2(omegai_bfrozen) -> omegai_bfrozen/1
  Bus Creator/1 -> Signal Conversion/1
  Signal Conversion/1 -> vortex parameters/1
  MATLAB Function1/4(p0_filament_left) -> Display/1, Bus Creator/1  "p0_filament_left"
  MATLAB Function1/5(p0_filament_right) -> Bus Creator/2  "p0_filament_right"
  MATLAB Function1/6(dcm_ew) -> Bus Creator/3  "dcm_ew"

== system formationFlyingBlockset/Cularis vortex geometry parameters ==
  Bus Creator : BusCreator  Inputs=9  OutDataTypeStr=Bus: VortexParameterBus  NonVirtualBus=on
  Constant : Constant  Value=uavsim.cularis.c
  Constant1 : Constant  Value=mask_ID
  Constant2 : Constant  Value=uavsim.cularis.b
  Constant3 : Constant  Value=uavsim.cularis.wingsweep_rad
  Constant4 : Constant  Value=uavsim.cularis.dihedral_rad
  Constant5 : Constant
  Constant6 : Constant  Value=[uavsim.cularis.c/2 0 0]
  Constant7 : Constant  Value=0.05
  Constant8 : Constant  Value=[0 0 -0.05]
  p : Outport
  wires:
  Constant8/1 -> Bus Creator/9  "posFinTip_b_m"
  Constant7/1 -> Bus Creator/8  "verticalRefLength_m"
  Constant6/1 -> Bus Creator/7  "pNose_b_m"
  Constant5/1 -> Bus Creator/6  "longiRefLength_m"
  Constant4/1 -> Bus Creator/5  "dihedral_rad"
  Constant3/1 -> Bus Creator/4  "sweep_rad"
  Constant2/1 -> Bus Creator/3  "b_m"
  Bus Creator/1 -> p/1
  Constant1/1 -> Bus Creator/2  "id"
  Constant/1 -> Bus Creator/1  "cbar_m"

== system formationFlyingBlockset/ECEF to flat earth ==
  X_ecef_m : Inport
  ECEF Position to LLA : aerolibtransform2/ECEF Position to LLA  units=Metric (MKS)  ptype=Earth (WGS84)  F=1/298.257223563  R=6378137
  LLA to Flat Earth : aerolibtransform2/LLA to Flat Earth  units=Metric (MKS)  ptype=Earth (WGS84)  F=1/298.257223563  R=6378137  LL0=rad2deg(mask_originNED_ECEF_rrm(1:2))  psi=0
  reference altitude of NED frame in ECEF frame : Constant  Value=mask_originNED_ECEF_rrm(3)
  X_ned_m : Outport
  wires:
  LLA to Flat Earth/1 -> X_ned_m/1
  X_ecef_m/1 -> ECEF Position to LLA/1
  ECEF Position to LLA/1 -> LLA to Flat Earth/1
  ECEF Position to LLA/2 -> LLA to Flat Earth/2
  reference altitude of NED frame in ECEF frame/1 -> LLA to Flat Earth/3

== system formationFlyingBlockset/Environment and terrain - turbulent wind - ==
  AirframeBus : Inport  OutDataTypeStr=Bus: Airframe
  Bus Selector4 : BusSelector  OutputSignals=Kinematics.Position.P_LLA_deg_m,Kinematics.Attitude.DCM_be,Aero.Va_mps
  Das muss so : Memory
  Environment turbulent wind : uavsimBlockset_Environment_turbulentWind/Environment turbulent wind  mask_constantwind_NED_mps=mask_ambientWind  mask_wingspan=mask_wingspan  mask_windON=mask_windON  mask_turbulenceON=1
  flat terrain : Constant  Value=0
  EnvDat : Outport  OutDataTypeStr=Bus: Environment
  wires:
  Das muss so/1 -> EnvDat/1
  Bus Selector4/1 -> Environment turbulent wind/1  "<P_LLA_deg_m>"
  AirframeBus/1 -> Bus Selector4/1
  Bus Selector4/2 -> Environment turbulent wind/3  "<DCM_be>"
  Bus Selector4/3 -> Environment turbulent wind/4  "<Va_mps>"
  flat terrain/1 -> Environment turbulent wind/2
  Environment turbulent wind/1 -> Das muss so/1

== system formationFlyingBlockset/Fixed wing avionics ==
  inter UAS com : Inport  OutDataTypeStr=Bus: iUAScom
  formation delta_p : Inport  Port=2
  true aircraft state : Inport  Port=3
  Environment : Inport  Port=4  OutDataTypeStr=Bus: Environment
  P propulsion : Inport  Port=5
  fstate_dx_in : Inport  Port=6
  vLeaderState : Inport  Port=7  OutDataTypeStr=Bus: iUAScom
  Add sensor errors : formationFlyingBlockset/Add sensor errors
  Bus Selector : BusSelector  OutputSignals=Kinematics.Position.P_NED_m,Kinematics.Velocity.Vground_NED_mps,Kinematics.Acceleration.VgroundDot_bfrozen_mps2,Kinematics.Attitude.DCM_be
  Command laws : Subsystem
  Display : Display
  Math Function : Math  Operator=transpose  SaturateOnIntegerOverflow=on
  Matrix Multiply : Product  Multiplication=Matrix(*)
  NED acceleration : formationFlyingBlockset/Signal to workspace  mask_id=['log_accNED_UAS' num2str(aircraftmask_ID) ]  mask_dt=0.01  mask_debug=log_accNED_UAS1
  NED position : formationFlyingBlockset/Signal to workspace  mask_id=['log_pNED_UAS' num2str(aircraftmask_ID) ]  mask_dt=0.1  mask_debug=log_pNED_UAS1
  NED velocity : formationFlyingBlockset/Signal to workspace  mask_id=['log_vNED_UAS' num2str(aircraftmask_ID) ]  mask_dt=0.1  mask_debug=log_vNED_UAS1
  PWM+computation delay : Delay  DelayLength=ceil(uavsim.avionics.totaltransportdelay_s/(1/uavsim.simConfig.sampleFrequency))
  Propulsion power : formationFlyingBlockset/Signal to workspace  mask_id=['log_P_propulsion_UAS' num2str(aircraftmask_ID) ]  mask_dt=0.1  mask_debug=log_P_propulsion_UAS1
  Sensor delays1 : Subsystem  Commented=on
  Sensor error models on/off : ManualSwitch
  Sensor log : formationFlyingBlockset/Signal to workspace  mask_id=['log_sensors_UAS' num2str(aircraftmask_ID) ]  mask_dt=0.01  mask_debug=log_sensors_UAS1
  Sensor log - error-free : formationFlyingBlockset/Signal to workspace  mask_id=['log_cleansensors_UAS' num2str(aircraftmask_ID) ]  mask_dt=0.01  mask_debug=log_cleansensors_UAS1
  Sensor package: error-free : formationFlyingBlockset/Sensor package: error-free
  State estimation department : formationFlyingBlockset/State estimation department
  u : Outport
  fstate_dx : Outport  Port=2
  wires:
  vLeaderState/1 -> Command laws/5(vLeaderState)
  Add sensor errors/1 -> Sensor error models on/off/2
  Sensor error models on/off/1 -> Sensor log/1, State estimation department/1
  Matrix Multiply/1 -> NED acceleration/1
  Math Function/1 -> Matrix Multiply/1
  Bus Selector/3 -> Matrix Multiply/2  "<VgroundDot_bfrozen_mps2>"
  Bus Selector/4 -> Math Function/1  "<DCM_be>"
  Command laws/1(u - system inputs) -> PWM+computation delay/1
  PWM+computation delay/1 -> u/1
  formation delta_p/1 -> Command laws/3(formationOffset_m)
  inter UAS com/1 -> Sensor package: error-free/2, Command laws/2(iUASCom)
  State estimation department/1 -> Command laws/1(Aircraft state estimate)
  Environment/1 -> Sensor package: error-free/3
  P propulsion/1 -> Propulsion power/1
  true aircraft state/1 -> Bus Selector/1, Sensor package: error-free/1
  Bus Selector/1 -> NED position/1  "<P_NED_m>"
  Bus Selector/2 -> NED velocity/1, Display/1  "<Vground_NED_mps>"
  Sensor package: error-free/1 -> Sensor log - error-free/1, Sensor error models on/off/1, Add sensor errors/1
  Command laws/2(fstate_dx) -> fstate_dx/1
  fstate_dx_in/1 -> Command laws/4(fstate_dx_in)

== system formationFlyingBlockset/Get p and v in LT frame ==
  v of LS frame in NED [mps] : Inport
  p NED   [m] : Inport  Port=2
  v NED [mps] : Inport  Port=3
  Constant : Constant  Value=zeros(2,1)
  Demux : Demux  Outputs=3
  Mux : Mux  Inputs=2
  Rotate position vector from NED to LS frame : Product  Multiplication=Matrix(*)
  Rotate velocity vector from NED to LS frame : Product  Multiplication=Matrix(*)
  Rotation Angles to Direction Cosine Matrix : aerolibtransform2/Rotation Angles to Direction Cosine Matrix  rotationOrder=ZYX
  Scope{1..3,5..6} (5 alike) : Scope
  Terminator1 : Terminator
  Trigonometric Function : Trigonometry  Operator=atan2
  p_LS : Outport
  v_LS : Outport  Port=2
  wires:
  Rotation Angles to Direction Cosine Matrix/1 -> Rotate velocity vector from NED to LS frame/1, Rotate position vector from NED to LS frame/1
  Demux/3 -> Terminator1/1
  Demux/1 -> Trigonometric Function/2
  Demux/2 -> Trigonometric Function/1
  v NED [mps]/1 -> Rotate velocity vector from NED to LS frame/2, Scope3/1
  Trigonometric Function/1 -> Mux/1
  Mux/1 -> Rotation Angles to Direction Cosine Matrix/1
  Constant/1 -> Mux/2
  p NED   [m]/1 -> Rotate position vector from NED to LS frame/2, Scope2/1
  Rotate position vector from NED to LS frame/1 -> p_LS/1, Scope6/1
  v of LS frame in NED [mps]/1 -> Demux/1, Scope1/1
  Rotate velocity vector from NED to LS frame/1 -> Scope5/1, v_LS/1

== system formationFlyingBlockset/Linear state observer ==
  y : Inport
  u : Inport  Port=2
  invC : Inport  Port=3
  D : Inport  Port=4
  Add : Sum
  Matrix Multiply : Product  Multiplication=Matrix(*)
  Matrix Multiply1 : Product  Multiplication=Matrix(*)
  Matrix Multiply2 : Product  Multiplication=Matrix(*)
  x : Outport
  wires:
  y/1 -> Matrix Multiply/2
  invC/1 -> Matrix Multiply1/1, Matrix Multiply/1
  D/1 -> Matrix Multiply1/2
  Matrix Multiply1/1 -> Matrix Multiply2/1
  u/1 -> Matrix Multiply2/2
  Matrix Multiply2/1 -> Add/2
  Matrix Multiply/1 -> Add/1
  Add/1 -> x/1
